simulink model "sysgenQAMExt"  (Simulink 7.7)
settings: Solver=ode45  StartTime=0.0  StopTime=3000  RelTol=1e-3
PreLoadFcn:
  | xlrequire('PreLoadFcn')
values from neighbouring files (symbols this model uses):
  hh = hh1/max(hh1)    [sysgenCostasLoop_PreLoadFcn.m]
  j = find(xLabel==')')    [sdspfscope2_r13.m]
  k = (k-1)*3+2    [sdspfscope2_r13.m]
  mu = xfix({xlSigned, 18, 15, xlRound, xlSaturate}, mu)    [lmsErr.m]
undefined symbols (not defined in the file or in its folder): chan, k_i0, k_p0, xlipgetpartsetting, xlsfunxy
libraries: xbsIndex_r4 x477, simulink x2, dspsigops x2, dspmlti4 x2, commchan3 x1, xbsCopyrightNotice_r4 x1, dspobslib x1
(part 1 of 5)
settings Model: Creator=alexc  LastModifiedBy=wayneh  ExtModeTrigMode=oneshot  ExtModeArmWhenConnect=off
settings DataIOCC: LimitDataPoints=off  SignalLoggingName=sigsOut
settings OptimizationCC: BlockReduction=off  BooleanDataType=off  InlineInvariantSignals=on  InitFltsAndDblsToZero=on
settings DebuggingCC: SaveWithParameterizedLinksMsg=none  SignalResolutionControl=TryResolveAllWithWarning  SolverPrmCheckMsg=none  MultiTaskDSMMsg=warning  MultiTaskCondExecSysMsg=none  StrictBusMsg=None
settings HardwareCC: TargetUnknown=on
settings RTWCC: IncludeERTFirstTime=on
settings GRTTargetCC: TargetFcnLib=ansi_tfl_tmw.mat

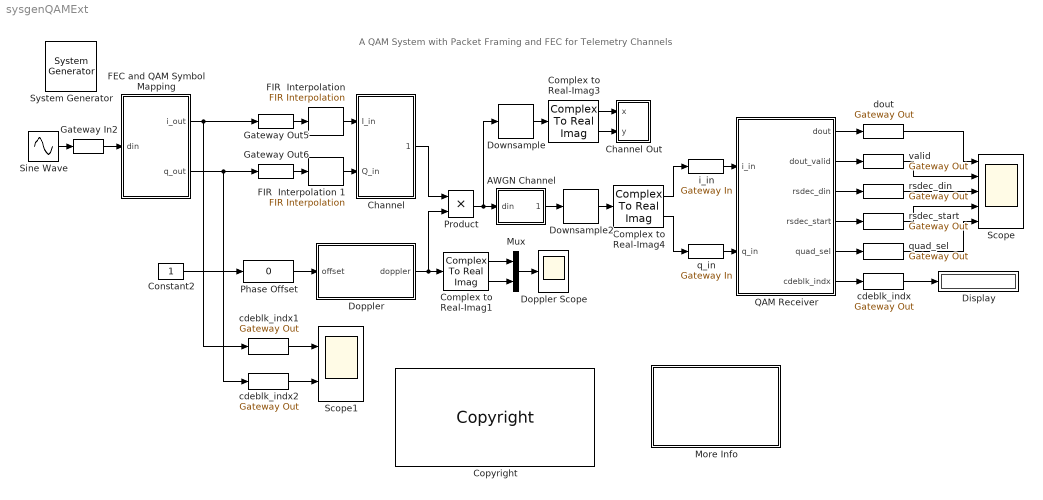
== system sysgenQAMExt ==
  note: A QAM System with Packet Framing and FEC for Telemetry Channels
  " System Generator" : xbsIndex_r4/ System Generator  Tag=genX  SystemSampleTime=-1  xilinxfamily=virtex6  part=xc6vlx240t  speed=-1  package=ff1156  synthesis_tool=XST  clock_wrapper=Clock Enables  directory=./netlist1  proj_type=Project Navigator  Synth_file=XST Defaults  Impl_file=ISE Defaults  testbench=off  simulink_period=1  sysclk_period=55  dcm_input_clock_period=100  incr_netlist=off  trim_vbits=Everywhere in SubSystem  dbl_ovrd=According to Block Masks  core_generation=According to Block Masks  run_coregen=off  deprecated_control=off  eval_field=0  block_type=sysgen
      settings: block_version=10.1.3
  AWGN Channel : Subsystem  mask{snr=4}
  Channel : Subsystem
  Channel Out : Subsystem  LoadFcn=xlsfunxy([],[],[],'LoadBlock')  StartFcn=xlsfunxy([],[],[],'Start')  StopFcn=xlsfunxy([],[],[],'Stop')  mask(My XY scope.){xmin=-2.25, xmax=2.25, ymin=-2.25, ymax=2.25, refresh=800, style='.', st=-1}
      mask prompts: xmin "x-min:"; xmax "x-max:"; ymin "y-min:"; ymax "y-max:"; refresh "Refresh rate"; style "Line/Marker style"; st "Sample time:"
      mask help: XY scope using MATLAB graph window. First input is used as time base. Enter plotting ranges.
      settings: CopyFcn=xlsfunxy([],[],[],'CopyBlock')  DeleteFcn=xlsfunxy([],[],[],'DeleteBlock')  NameChangeFcn=xlsfunxy([],[],[],'NameChange')
      mask Help: This block can be used to explore limit cycles. Look at the m-file xlsfunxy.m to see how it works.
      mask Display: plot([.05 .95 .95 .05 .05],[.45 .45 .95 .95 .45], 0.5+cos(0:0.1:2*pi)*0.3,0.7+sin(0:0.1:2*pi)*0.2)
  Complex to Real-Imag1 : ComplexToRealImag
  Complex to Real-Imag3 : ComplexToRealImag
  Complex to Real-Imag4 : ComplexToRealImag
  Constant2 : Constant
  Copyright : xbsCopyrightNotice_r4/Copyright  copyrighttext="Copyright (c) 2011  by  Xilinx, Inc. All rights reserved.<br><br>This file contains proprietary, confidential information of Xilinx, Inc., is distributed under license from Xilinx, Inc., and may be used, copied and/or disclosed only pursuant to the terms of a valid license agreement with Xilinx, Inc. Xilinx hereby grants you a license to use this file solely for design, simulation, implementation and creation of design files limited to Xilinx devices or technologies. Use with non-Xilinx devices or technologies is expressly prohibited and immediately terminates your license unless covered by a separate agreement.<br><br>Xilinx is providing this design, code, or information \"as-is\" solely for use in developing programs and solutions for Xilinx devices, with no obligation on the part of Xilinx to provide support. By providing this design, code, or information as one possible implementation of this feature, application or standard, Xilinx is making no representation that this implementation is free from any claims of infringement. You are responsible for obtaining any rights you may require for your implementation. Xilinx expressly disclaims any warranty whatsoever with respect to the adequacy of the implementation, including but not limited to any warranties or representations that this implementation is free from claims of infringement, implied warranties of merchantability or fitness for a particular purpose.<br><br>Xilinx products are not intended for use in life support appliances, devices, or systems. Use in such applications is expressly prohibited.<br><br>Any modifications that are made to the Source Code are done at the user's sole risk and will be unsupported.<br><br>This copyright and support notice must be retained as part of this text at all times. (c) Copyright 1995-2011 Xilinx, Inc. All rights reserved."  block_type=copyright
      settings: block_version=10.1.00
      settings: infoedit=|
      | Copyright(C) 2008 by  Xilinx, Inc. All rights reserved.<br>
      | <br>
      | This file contains proprietary, confidential information of Xilinx, Inc., is distributed under license
      | from Xilinx, Inc., and may be used, copied and/or disclosed only pursuant to the terms of a valid license
      | agreement with Xilinx, Inc. Xilinx hereby grants you a license to use this file solely for design,
      | simulation, implementation and creation of design files limited to Xilinx devices or technologies. Use
      | with non-Xilinx devices or technologies is expressly prohibited and immediately terminates your license
      | unless covered by a separate agreement.<br>
      | <br>
      | Xilinx is providing this design, code, or information "as-is" solely for use in developing programs and
      | solutions for Xilinx devices, with no obligation on the part of Xilinx to provide support. By providing
      | this design, code, or information as one possible implementation of this feature, application or standard,
      | Xilinx is making no representation that this implementation is free from any claims of infringement. You
      | are responsible for obtaining any rights you may require for your implementation. Xilinx expressly disclaims
      | any warranty whatsoever with respect to the adequacy of the implementation, including but not limited to any
      | warranties or representations that this implementation is free from claims of infringement, implied warranties
      | of merchantability or fitness for a particular purpose.<br>
      | <br>
      | Xilinx products are not intended for use in life support appliances, devices, or systems. Use in such
      | applications is expressly prohibited.<br>
      | <br>
      | Any modifications that are made to the Source Code are done at the user's sole risk and will be unsupported.<br>
      | <br>
      | This copyright and support notice must be retained as part of this text at all times.
      | (c) Copyright 1995-2008 Xilinx, Inc. All rights reserved.
  Display : Display
  Doppler : Subsystem
  Doppler Scope : Scope
      settings: TimeRange=4000  YMin=-0.6  YMax=1
  Downsample : dspsigops/Downsample  N=4  phase=0  InputProcessing=Inherited (this choice will be removed - see release notes)  RateOptions=Enforce single-rate processing  smode=Allow multirate  fmode=Maintain input frame size  ic=0
  Downsample2 : dspsigops/Downsample  N=2  phase=0  InputProcessing=Inherited (this choice will be removed - see release notes)  RateOptions=Enforce single-rate processing  smode=Allow multirate  fmode=Maintain input frame size  ic=0
  FEC and QAM Symbol Mapping : Subsystem
  "FIR  Interpolation " : dspmlti4/FIR Interpolation  h=[hh]  L=4  framing=Maintain input frame size  outputBufInitCond=0  InputProcessing=Inherited (this choice will be removed - see release notes)  firstCoeffDataTypeStr=Inherit: Same word length as input  firstCoeffLastDataTypeStr=Inherit: Same word length as input  firstCoeffMin=[]  firstCoeffMax=[]  outputDataTypeStr=Inherit: Same as accumulator  outputLastDataTypeStr=Inherit: Same as accumulator  outputMin=[]  outputMax=[]  roundingMode=Floor  overflowMode=off  FilterSource=Specify via dialog  FilterObject=Hm_firinterp
  FIR  Interpolation 1 : dspmlti4/FIR Interpolation  h=[hh]  L=4  framing=Maintain input frame size  outputBufInitCond=0  InputProcessing=Inherited (this choice will be removed - see release notes)  firstCoeffDataTypeStr=Inherit: Same word length as input  firstCoeffLastDataTypeStr=Inherit: Same word length as input  firstCoeffMin=[]  firstCoeffMax=[]  outputDataTypeStr=Inherit: Same as accumulator  outputLastDataTypeStr=Inherit: Same as accumulator  outputMin=[]  outputMax=[]  roundingMode=Floor  overflowMode=off  FilterSource=Specify via dialog  FilterObject=Hm_firinterp
  Gateway In2 : xbsIndex_r4/Gateway In  gui_display_data_type=Fixed-point  arith_type="Signed  (2's comp)"  n_bits=8  bin_pt=7  preci_type=Single  exp_width=8  frac_width=24  quantization="Round  (unbiased: +/- Inf)"  overflow=Saturate  period=16  dbl_ovrd=off  timing_constraint=None  locs_specified=off  LOCs={}  inherit_from_input=off  UseAsADC=off  ADCChannel='1'  hdl_port=on  block_type=gatewayin
      settings: infoedit="Gateway in block.  Converts inputs of type Simulink integer, double and fixed point to  Xilinx fixed point type.<P><P>Hardware notes:  In hardware these blocks become top level input ports."  xl_area=[0, 0, 0, 0, 0, 0, 0]  block_version=VER_STRING_GOES_HERE
  Gateway Out5 : xbsIndex_r4/Gateway Out  inherit_from_input=off  hdl_port=on  timing_constraint=None  locs_specified=off  LOCs={}  UseAsDAC=off  DACChannel='1'  block_type=gatewayout
      settings: infoedit="Gateway out block.  Converts Xilinx fixed point inputs into ouputs of type Simulink integer, double, or fixed point.<P><P>Hardware notes:  In hardware these blocks become top level output ports or are discarded, depending on how they are configured."  xl_area=[0, 0, 0, 0, 0, 0, 0]  block_version=VER_STRING_GOES_HERE
  Gateway Out6 : xbsIndex_r4/Gateway Out  inherit_from_input=off  hdl_port=on  timing_constraint=None  locs_specified=off  LOCs={}  UseAsDAC=off  DACChannel='1'  block_type=gatewayout
      settings: infoedit="Gateway out block.  Converts Xilinx fixed point inputs into ouputs of type Simulink integer, double, or fixed point.<P><P>Hardware notes:  In hardware these blocks become top level output ports or are discarded, depending on how they are configured."  xl_area=[0, 0, 0, 0, 0, 0, 0]  block_version=VER_STRING_GOES_HERE
  More Info : Subsystem
      mask Display: disp('Double click\n for\n more information.')
  Mux : Mux  Inputs=2
  Phase Offset : simulink/Math Operations/Slider Gain  SystemSampleTime=-1  low=0  gain=0  high=1
  Product : Product  SaturateOnIntegerOverflow=on  InputSameDT=on  OutDataTypeStr=Inherit: Same as first input
  QAM Receiver : Subsystem
  Scope : Scope  NumInputPorts=5
      settings: TimeRange=5000  YMin=-1~-1~-1~-1~-1  YMax=1~1~1~1~1
  Scope1 : Scope  NumInputPorts=2
      settings: TimeRange=10000  YMin=-1~-1  YMax=1~1  SaveName=ScopeData2
  Sine Wave : Sin  Frequency=1/255  SampleTime=16
  cdeblk_indx : xbsIndex_r4/Gateway Out  inherit_from_input=off  hdl_port=on  timing_constraint=None  locs_specified=off  LOCs={}  UseAsDAC=off  DACChannel='1'  block_type=gatewayout
      settings: infoedit="Gateway out block.  Converts Xilinx fixed point inputs into ouputs of type Simulink integer, double, or fixed point.<P><P>Hardware notes:  In hardware these blocks become top level output ports or are discarded, depending on how they are configured."  xl_area=[0, 0, 0, 0, 0, 0, 0]  block_version=VER_STRING_GOES_HERE
  cdeblk_indx1 : xbsIndex_r4/Gateway Out  inherit_from_input=off  hdl_port=off  timing_constraint=None  locs_specified=off  LOCs={}  UseAsDAC=off  DACChannel='1'  block_type=gatewayout
      settings: infoedit="Gateway out block.  Converts Xilinx fixed point inputs into ouputs of type Simulink integer, double, or fixed point.<br><br>Hardware notes:  In hardware these blocks become top level output ports or are discarded, depending on how they are configured."  xl_area=[0, 0, 0, 0, 0, 0, 0]  block_version=VER_STRING_GOES_HERE
  cdeblk_indx2 : xbsIndex_r4/Gateway Out  inherit_from_input=off  hdl_port=off  timing_constraint=None  locs_specified=off  LOCs={}  UseAsDAC=off  DACChannel='1'  block_type=gatewayout
      settings: infoedit="Gateway out block.  Converts Xilinx fixed point inputs into ouputs of type Simulink integer, double, or fixed point.<br><br>Hardware notes:  In hardware these blocks become top level output ports or are discarded, depending on how they are configured."  xl_area=[0, 0, 0, 0, 0, 0, 0]  block_version=VER_STRING_GOES_HERE
  dout : xbsIndex_r4/Gateway Out  inherit_from_input=off  hdl_port=on  timing_constraint=None  locs_specified=off  LOCs={}  UseAsDAC=off  DACChannel='1'  block_type=gatewayout
      settings: infoedit="Gateway out block.  Converts Xilinx fixed point inputs into ouputs of type Simulink integer, double, or fixed point.<P><P>Hardware notes:  In hardware these blocks become top level output ports or are discarded, depending on how they are configured."  xl_area=[0, 0, 0, 0, 0, 0, 0]  block_version=VER_STRING_GOES_HERE
  i_in : xbsIndex_r4/Gateway In  gui_display_data_type=Fixed-point  arith_type="Signed  (2's comp)"  n_bits=xn_ni  bin_pt=xn_nf  preci_type=Single  exp_width=8  frac_width=24  quantization="Round  (unbiased: +/- Inf)"  overflow=Saturate  period=2  dbl_ovrd=off  timing_constraint=None  locs_specified=off  LOCs={}  inherit_from_input=off  UseAsADC=off  ADCChannel='1'  hdl_port=on  block_type=gatewayin
      settings: infoedit="Gateway in block.  Converts inputs of type Simulink integer, double and fixed point to  Xilinx fixed point type.<P><P>Hardware notes:  In hardware these blocks become top level input ports."  xl_area=[0, 0, 0, 0, 0, 0, 0]  block_version=VER_STRING_GOES_HERE
  q_in : xbsIndex_r4/Gateway In  gui_display_data_type=Fixed-point  arith_type="Signed  (2's comp)"  n_bits=xn_ni  bin_pt=xn_nf  preci_type=Single  exp_width=8  frac_width=24  quantization="Round  (unbiased: +/- Inf)"  overflow=Saturate  period=2  dbl_ovrd=off  timing_constraint=None  locs_specified=off  LOCs={}  inherit_from_input=off  UseAsADC=off  ADCChannel='1'  hdl_port=on  block_type=gatewayin
      settings: infoedit="Gateway in block.  Converts inputs of type Simulink integer, double and fixed point to  Xilinx fixed point type.<P><P>Hardware notes:  In hardware these blocks become top level input ports."  xl_area=[0, 0, 0, 0, 0, 0, 0]  block_version=VER_STRING_GOES_HERE
  quad_sel : xbsIndex_r4/Gateway Out  inherit_from_input=off  hdl_port=on  timing_constraint=None  locs_specified=off  LOCs={}  UseAsDAC=off  DACChannel='1'  block_type=gatewayout
      settings: infoedit="Gateway out block.  Converts Xilinx fixed point inputs into ouputs of type Simulink integer, double, or fixed point.<P><P>Hardware notes:  In hardware these blocks become top level output ports or are discarded, depending on how they are configured."  xl_area=[0, 0, 0, 0, 0, 0, 0]  block_version=VER_STRING_GOES_HERE
  rsdec_din : xbsIndex_r4/Gateway Out  inherit_from_input=off  hdl_port=on  timing_constraint=None  locs_specified=off  LOCs={}  UseAsDAC=off  DACChannel='1'  block_type=gatewayout
      settings: infoedit="Gateway out block.  Converts Xilinx fixed point inputs into ouputs of type Simulink integer, double, or fixed point.<P><P>Hardware notes:  In hardware these blocks become top level output ports or are discarded, depending on how they are configured."  xl_area=[0, 0, 0, 0, 0, 0, 0]  block_version=VER_STRING_GOES_HERE
  rsdec_start : xbsIndex_r4/Gateway Out  inherit_from_input=off  hdl_port=on  timing_constraint=None  locs_specified=off  LOCs={}  UseAsDAC=off  DACChannel='1'  block_type=gatewayout
      settings: infoedit="Gateway out block.  Converts Xilinx fixed point inputs into ouputs of type Simulink integer, double, or fixed point.<P><P>Hardware notes:  In hardware these blocks become top level output ports or are discarded, depending on how they are configured."  xl_area=[0, 0, 0, 0, 0, 0, 0]  block_version=VER_STRING_GOES_HERE
  valid : xbsIndex_r4/Gateway Out  inherit_from_input=off  hdl_port=on  timing_constraint=None  locs_specified=off  LOCs={}  UseAsDAC=off  DACChannel='1'  block_type=gatewayout
      settings: infoedit="Gateway out block.  Converts Xilinx fixed point inputs into ouputs of type Simulink integer, double, or fixed point.<P><P>Hardware notes:  In hardware these blocks become top level output ports or are discarded, depending on how they are configured."  xl_area=[0, 0, 0, 0, 0, 0, 0]  block_version=VER_STRING_GOES_HERE
  wires:
  FEC and QAM Symbol Mapping/1(i_out) -> Gateway Out5/1, cdeblk_indx1/1
  FEC and QAM Symbol Mapping/2(q_out) -> Gateway Out6/1, cdeblk_indx2/1
  Channel/1(chan_out) -> Product/1
  Doppler/1(doppler) -> Product/2, Complex to Real-Imag1/1
  i_in/1 -> QAM Receiver/1(i_in)
  q_in/1 -> QAM Receiver/2(q_in)
  Product/1 -> AWGN Channel/1(din), Downsample/1
  Phase Offset/1 -> Doppler/1(offset)
  Constant2/1 -> Phase Offset/1
  Mux/1 -> Doppler Scope/1
  Complex to Real-Imag1/1 -> Mux/1
  Complex to Real-Imag1/2 -> Mux/2
  cdeblk_indx/1 -> Display/1
  QAM Receiver/6(cdeblk_indx) -> cdeblk_indx/1
  Downsample2/1 -> Complex to Real-Imag4/1
  Complex to Real-Imag4/2 -> q_in/1
  Complex to Real-Imag4/1 -> i_in/1
  Downsample/1 -> Complex to Real-Imag3/1
  Complex to Real-Imag3/2 -> Channel Out/2(y)
  Complex to Real-Imag3/1 -> Channel Out/1(x)
  "FIR  Interpolation "/1 -> Channel/1(I_in)
  FIR  Interpolation 1/1 -> Channel/2(Q_in)
  Gateway Out5/1 -> "FIR  Interpolation "/1
  Gateway Out6/1 -> FIR  Interpolation 1/1
  Sine Wave/1 -> Gateway In2/1
  Gateway In2/1 -> FEC and QAM Symbol Mapping/1(din)
  AWGN Channel/1(dout) -> Downsample2/1
  QAM Receiver/1(dout) -> dout/1
  QAM Receiver/2(dout_valid) -> valid/1
  QAM Receiver/3(rsdec_din) -> rsdec_din/1
  QAM Receiver/5(quad_sel) -> quad_sel/1
  QAM Receiver/4(rsdec_start) -> rsdec_start/1
  quad_sel/1 -> Scope/5
  rsdec_din/1 -> Scope/3
  rsdec_start/1 -> Scope/4
  dout/1 -> Scope/1
  valid/1 -> Scope/2
  cdeblk_indx1/1 -> Scope1/1
  cdeblk_indx2/1 -> Scope1/2

== system sysgenQAMExt/AWGN Channel ==
  din : Inport
  AWGN Channel : commchan3/AWGN Channel  SystemSampleTime=-1  InputProcessing=Inherited (this choice will be removed - see release notes)  seed=54321  noiseMode="Signal to noise ratio  (SNR)"  EbNodB=10  EsNodB=10  SNRdB=snr  bitsPerSym=1  Ps=1/16  Tsym=1  variance=1
  dout : Outport
  wires:
  AWGN Channel/1 -> dout/1
  din/1 -> AWGN Channel/1

== system sysgenQAMExt/Channel ==
  I_in : Inport
  Q_in : Inport  Port=2
  Channel : Subsystem
  Channel1 : Subsystem
  Gain : Gain  Gain=j  SaturateOnIntegerOverflow=on  OutDataTypeStr=Inherit: Same as input  ParamDataTypeStr=Inherit: Same as input
  Sum : Sum  SaturateOnIntegerOverflow=on  InputSameDT=on  OutDataTypeStr=Inherit: Same as first input
  chan_out : Outport
  wires:
  Gain/1 -> Sum/2
  Channel/1(y_n) -> Sum/1
  Channel1/1(y_n) -> Gain/1
  I_in/1 -> Channel/1(x_n)
  Q_in/1 -> Channel1/1(x_n)
  Sum/1 -> chan_out/1

== system sysgenQAMExt/Channel Out ==
  x : Inport
  y : Inport  Port=2
  Mux : Mux  Inputs=2
  xlsfunxy : S-Function  FunctionName=xlsfunxy  Parameters=[xmin xmax ymin ymax],refresh,style,st  EnableBusSupport=off
  wires:
  Mux/1 -> xlsfunxy/1
  x/1 -> Mux/1
  y/1 -> Mux/2

== system sysgenQAMExt/Doppler ==
  offset : Inport
  DSP Constant : dspobslib/DSP Constant  SystemSampleTime=-1  Value=1  SampleMode=Discrete  discreteOutput=Sample-based  continuousOutput=Sample-based  sampTime=1  framePeriod=1  dataType=Inherit from 'Constant value'  isSigned=on  wordLen=16  udDataType=sfix(16)  fracBitsMode=Best precision  numFracBits=15  InterpretAs1D=off  Ts=1  FramebasedOutput=off
  Frequency Delta : simulink/Math Operations/Slider Gain  SystemSampleTime=-1  low=-0.1  gain=0.001  high=0.1
  R:I : RealImagToComplex
  TX Doppler : Subsystem
  Terminator : Terminator
  doppler : Outport
  wires:
  TX Doppler/1(Cos) -> R:I/1
  TX Doppler/2(Sin) -> R:I/2
  DSP Constant/1 -> Frequency Delta/1
  R:I/1 -> doppler/1
  TX Doppler/3(DDS Theta) -> Terminator/1
  Frequency Delta/1 -> TX Doppler/1(In1)
  offset/1 -> TX Doppler/2(Phase Offset)

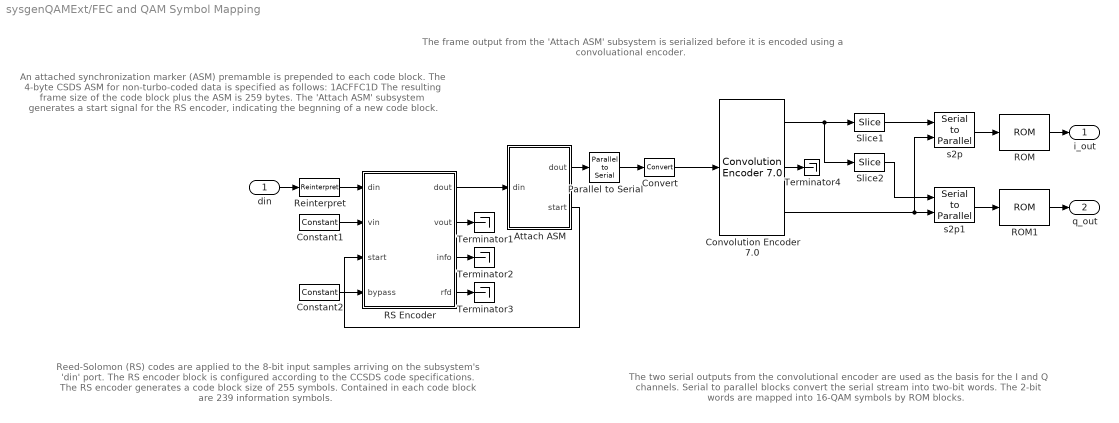
== system sysgenQAMExt/FEC and QAM Symbol Mapping ==
  note: Reed-Solomon (RS) codes are applied to the 8-bit input samples
      | arriving on the subsystem's 'din' port.  The RS encoder block is
      | configured according to the CCSDS code specifications.  The RS
      | encoder generates a code block size of 255 symbols.  Contained
      | in each code block are 239 information symbols.
  note: An attached synchronization marker (ASM) premamble
      | is prepended to each code block.  The 4-byte CSDS
      | ASM for non-turbo-coded data is specified as follows:
      |
      | 1ACFFC1D
      |
      | The resulting frame size of the code block plus the ASM
      | is  259 bytes.  The 'Attach ASM' subsystem generates a
      | start signal for the RS encoder, indicating the begnning
      | of a new code block.
  note: The frame output from the 'Attach ASM' subsystem is serialized
      | before it is encoded using a convoluational encoder.
  note: The two serial outputs from the convolutional
      | encoder are used as the basis for the I and Q
      | channels.  Serial to parallel blocks convert the
      | serial stream into two-bit words.
      |
      | The 2-bit words are mapped into 16-QAM
      | symbols by ROM blocks.
  din : Inport
  Attach ASM : Subsystem
  Constant1 : xbsIndex_r4/Constant  const=1  gui_display_data_type=Fixed-point  arith_type=Boolean  n_bits=1  bin_pt=0  preci_type=Single  exp_width=8  frac_width=24  explicit_period=off  period=1  equ=P=C  opselect=C  inp2=PCIN>>17  opr=+  inp1=P  carry=CIN  dbl_ovrd=off  block_type=constant
      settings: block_version=VER_STRING_GOES_HERE
  Constant2 : xbsIndex_r4/Constant  const=0  gui_display_data_type=Fixed-point  arith_type=Boolean  n_bits=1  bin_pt=0  preci_type=Single  exp_width=8  frac_width=24  explicit_period=off  period=1  equ=P=C  opselect=C  inp2=PCIN>>17  opr=+  inp1=P  carry=CIN  dbl_ovrd=off  block_type=constant
      settings: block_version=VER_STRING_GOES_HERE
  Convert : xbsIndex_r4/Convert  gui_display_data_type=Fixed-point  arith_type=Boolean  n_bits=16  bin_pt=14  float_type=Single  exp_bits=8  fraction_bits=24  quantization=Truncate  overflow=Wrap  en=off  latency=0  dbl_ovrd=off  pipeline=off  block_type=convert
      settings: block_version=11.4
  "Convolution Encoder 7.0 " : xbsIndex_r4/Convolution Encoder 7.0   input_rate=1  output_rate=2  punctured=off  dual_output=off  puncture_code0='0'  puncture_code1='0'  constraint_length=7  convolution_code0='1111001'  convolution_code1='1011011'  convolution_code2='0000011'  convolution_code3='0000011'  convolution_code4='0000011'  convolution_code5='0000011'  convolution_code6='0000011'  nd=off  rfd=on  fd_in=off  rffd=off  rdy=on  synchronous_clear=off  ce=off  ip_name=Convolution Encoder  ip_version=7.0  dsptool_ready=false  ipcore_usecache=true  ipcore_useipmodelcache=true  wrapper_available=true  port_translation_map={ 'ce' => 'en', 'sclr' => 'rst'}  structural_sim=true  ipcore_do_not_force_period=true  block_type=convolution_v7_0
      settings: block_version=11.4
  Parallel to Serial : xbsIndex_r4/Parallel to Serial  output_order=Most Significant Word First  arith_type=Unsigned  output_bits=1  bin_pt=0  rst=off  en=off  latency=0  dbl_ovrd=off  block_type=p2s
      settings: infoedit=Each sample presented at the input becomes several samples presented serially at the output.  xl_area=[0, 0, 0, 0, 0, 0, 0]  block_version=VER_STRING_GOES_HERE
  ROM : xbsIndex_r4/ROM  depth=4  initVector=[1/3 1 -1/3 -1]  distributed_mem=Block RAM  rst=off  init_reg=0  en=off  latency=1  gui_display_data_type=Fixed-point  arith_type="Signed  (2's comp)"  n_bits=16  bin_pt=15  preci_type=Single  exp_width=8  frac_width=24  dbl_ovrd=off  optimize=Area  use_rpm=off  block_type=sprom
      settings: xl_area=[0, 0, 0, 0, 0, 0, 0]  block_version=VER_STRING_GOES_HERE
  ROM1 : xbsIndex_r4/ROM  depth=4  initVector=[1/3 1 -1/3 -1]  distributed_mem=Block RAM  rst=off  init_reg=0  en=off  latency=1  gui_display_data_type=Fixed-point  arith_type="Signed  (2's comp)"  n_bits=16  bin_pt=15  preci_type=Single  exp_width=8  frac_width=24  dbl_ovrd=off  optimize=Area  use_rpm=off  block_type=sprom
      settings: xl_area=[0, 0, 0, 0, 0, 0, 0]  block_version=VER_STRING_GOES_HERE
  RS Encoder : Subsystem
      settings: CopyFcn=set_param(gcb, 'LinkStatus', 'none');
  Reinterpret : xbsIndex_r4/Reinterpret  force_arith_type=on  arith_type=Unsigned  force_bin_pt=on  bin_pt=0  block_type=cast
      settings: infoedit="Changes type of samples without altering their binary representation.<P><P>Hardware notes: In hardware this block costs nothing.<P><P>Example:  Suppose the input is 6 bits wide, signed, with 2 fractional bits, and the output is forced to unsigned with 0 fractional bits.  Then an input of -2.0 (1110.00 in binary 2's complement) becomes an output of 56 (111000 in binary)."  block_version=VER_STRING_GOES_HERE
  Slice1 : xbsIndex_r4/Slice  nbits=1  boolean_output=off  mode=Lower Bit Location + Width  bit1=0  base1=MSB of Input  bit0=0  base0=LSB of Input  dbl_ovrd=off  block_type=slice
  Slice2 : xbsIndex_r4/Slice  nbits=1  boolean_output=off  mode=Upper Bit Location + Width  bit1=0  base1=MSB of Input  bit0=0  base0=LSB of Input  dbl_ovrd=off  block_type=slice
  Terminator{1..4} (4 alike) : Terminator
  s2p : xbsIndex_r4/Serial to Parallel  input_order=Least Significant Word First  arith_type=Unsigned  output_bits=2  bin_pt=0  rst=off  en=on  latency=1  dbl_ovrd=off  block_type=s2p
      settings: infoedit=Groups of samples presented serially at the input become single samples presented at the output.  xl_area=[0, 0, 0, 0, 0, 0, 0]  block_version=VER_STRING_GOES_HERE
  s2p1 : xbsIndex_r4/Serial to Parallel  input_order=Least Significant Word First  arith_type=Unsigned  output_bits=2  bin_pt=0  rst=off  en=on  latency=1  dbl_ovrd=off  block_type=s2p
      settings: infoedit=Groups of samples presented serially at the input become single samples presented at the output.  xl_area=[0, 0, 0, 0, 0, 0, 0]  block_version=VER_STRING_GOES_HERE
  i_out : Outport
  q_out : Outport  Port=2
  wires:
  ROM/1 -> i_out/1
  ROM1/1 -> q_out/1
  "Convolution Encoder 7.0 "/1 -> Slice1/1, Slice2/1
  s2p/1 -> ROM/1
  s2p1/1 -> ROM1/1
  Parallel to Serial/1 -> Convert/1
  Attach ASM/1(dout) -> Parallel to Serial/1
  din/1 -> Reinterpret/1
  RS Encoder/1(dout) -> Attach ASM/1(din)
  Constant1/1 -> RS Encoder/2(vin)
  Constant2/1 -> RS Encoder/4(bypass)
  Attach ASM/2(start) -> RS Encoder/3(start)
  Reinterpret/1 -> RS Encoder/1(din)
  RS Encoder/2(vout) -> Terminator1/1
  RS Encoder/3(info) -> Terminator2/1
  RS Encoder/4(rfd) -> Terminator3/1
  Convert/1 -> "Convolution Encoder 7.0 "/1
  Slice1/1 -> s2p/1
  Slice2/1 -> s2p1/1
  "Convolution Encoder 7.0 "/3 -> s2p1/2, s2p/2
  "Convolution Encoder 7.0 "/2 -> Terminator4/1

== system sysgenQAMExt/More Info ==
  note: A QAM System with Packet Framing and FEC for Telemetry Channels
  note: This design implements a QAM system with packet framing and FEC for telemetry channels.
      | The system is implemented according to the specifications provided by the Consultative
      | Committee for Space Data Systems for telemetry channel coding specification
      | (CCSDS 101.0-B-5).
      |
      | A sinusoidal source provides 8-bit samples to the 'FEC and QAM Symbol Mapping' subsystem.
      | Forward Error Correction (FEC) is applied to the samples and an attached synchronization
      | marker (ASM) is asserted at the start of each code block.   The data is mapped into 16-QAM
      | symbols and then interpolated.  Doppler content, ISI, and white Guassian noise are introduced
      | into the signal before it enters the receiver subsystem.
      |
      | The receiver employs a 16-QAM demodulator that performs adaptive channel equalization
      | and carrier recovery on a QAM input source.  The ASM is stripped from the demodulated data
      | before concatenated FEC is applied.  A PicoBlaze microcontroller controls the RS decoder,
      | maintains frame alignment of the received packects, and performs periodic adjustments of
      | the de-mapping QAM-16 quadrant reference.
      |
      | The CCSDS specification document can be found at the following URL:
      | http://nssdcftp.gsfc.nasa.gov/standards/ccsds/pdf/CCSDS-101.0-B-5.pdf
      |
      | For more information on the 16-QAM demodulator implementation and FPGA software-defined radios
      | in general, consult the following references:
      |
      | Chris H. Dick and Fred Harris, "FPGA QAM Demodulator Design," Field Programmable Logic
      | Conference (FPL), Sept. 2-4 Montpellier, France, 2002.
      |
      | Chris H. Dick, "Design and implementation of high-performance FPGA signal processing
      | datapaths for software-defined radios" VMEbus Systems, August 2001

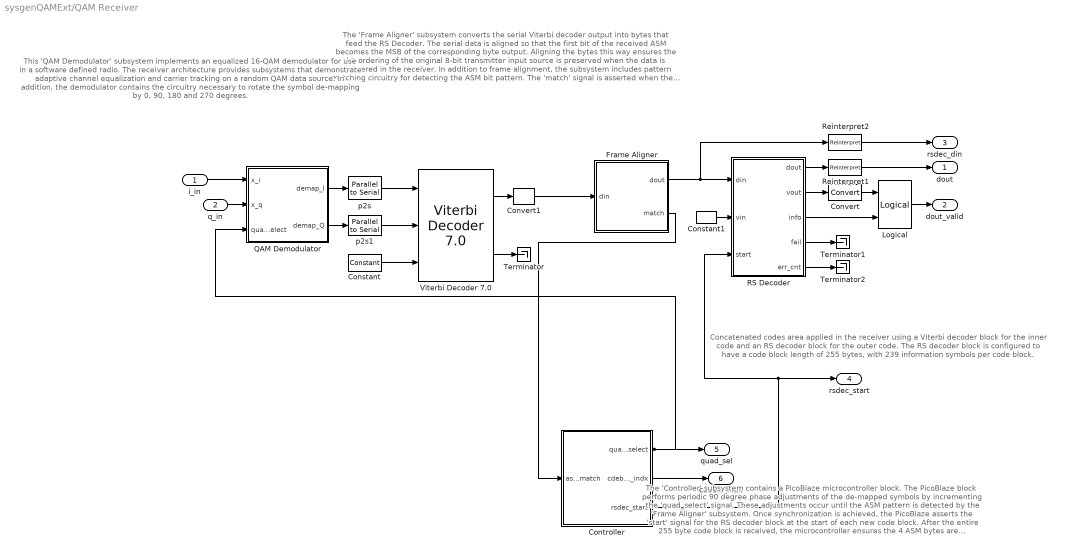
== system sysgenQAMExt/QAM Receiver ==
  note: The 'Frame Aligner' subsystem converts the serial Viterbi decoder output
      | into bytes that feed the RS Decoder.  The serial data is aligned so that the
      | first bit of the received ASM  becomes the MSB of the corresponding byte
      | output.  Aligning the bytes this way ensures the bit ordering of the original
      | 8-bit transmitter input source is preserved when the data is recovered in the
      | receiver.
      |
      | In addition to frame alignment, the subsystem includes pattern matching
      | circuitry for detecting the ASM bit pattern. The 'match' signal is asserted
      | when the ASM is detected.  The match signal is asserted when the last
      | byte of the ASM is presented on the 'dout' port.
  note: The 'Controller' subsystem contains a PicoBlaze microcontroller block.
      | The PicoBlaze block performs periodic 90 degree phase adjustments of
      | the de-mapped symbols by incrementing the 'quad_select' signal.
      | These adjustments occur until the ASM pattern is detected by the 'Frame
      | Aligner' subsystem.
      |
      | Once synchronization is achieved, the PicoBlaze asserts the 'start' signal
      | for the RS decoder block at the start of each new code block.  After the
      | entire 255 byte code block is received, the microcontroller ensures the 4
      | ASM bytes are successfully detected in the frame aligner.
      |
      | If synchronization is lost, i.e. the ASM is not detected, the microcontroller
      | will continue making adjustments to the 'quad_select' signal until the ASM
      | is once again detected.
  note: This 'QAM Demodulator' subsystem implements an equalized 16-QAM
      | demodulator for use in a software defined radio.  The receiver
      | architecture provides subsystems that demonstrate adaptive channel
      | equalization and carrier tracking on a random QAM data source.  In
      | addition, the demodulator contains the circuitry necessary to rotate the
      | symbol de-mapping by 0, 90, 180 and 270 degrees.
  note: Concatenated codes area applied in the receiver
      | using a Viterbi decoder block for the inner code
      | and an RS decoder block for the outer code.  The
      | RS decoder block is configured to have a code
      | block length of 255 bytes, with 239 information
      | symbols per code block.
  i_in : Inport
  q_in : Inport  Port=2
  Constant : xbsIndex_r4/Constant  const=1  gui_display_data_type=Fixed-point  arith_type=Boolean  n_bits=1  bin_pt=0  preci_type=Single  exp_width=8  frac_width=24  explicit_period=off  period=1  equ=P=C  opselect=C  inp2=PCIN>>17  opr=+  inp1=P  carry=CIN  dbl_ovrd=off  block_type=constant
      settings: block_version=VER_STRING_GOES_HERE
  Constant1 : xbsIndex_r4/Constant  const=1  gui_display_data_type=Fixed-point  arith_type=Boolean  n_bits=1  bin_pt=0  preci_type=Single  exp_width=8  frac_width=24  explicit_period=off  period=1  equ=P=C  opselect=C  inp2=PCIN>>17  opr=+  inp1=P  carry=CIN  dbl_ovrd=off  block_type=constant
      settings: block_version=VER_STRING_GOES_HERE
  Controller : Subsystem
  Convert : xbsIndex_r4/Convert  gui_display_data_type=Fixed-point  arith_type=Unsigned  n_bits=1  bin_pt=0  float_type=Single  exp_bits=8  fraction_bits=24  quantization=Truncate  overflow=Wrap  en=off  latency=0  dbl_ovrd=off  pipeline=off  block_type=convert
      settings: infoedit=The input is presented at the output after quantization and overflow effects.<P><P>Hardware notes: Additional hardware is used when rounding or saturation is selected and output width is less than the input width.  xl_area=[0, 0, 0, 0, 0, 0, 0]  block_version=VER_STRING_GOES_HERE
  Convert1 : xbsIndex_r4/Convert  gui_display_data_type=Fixed-point  arith_type=Unsigned  n_bits=1  bin_pt=0  float_type=Single  exp_bits=8  fraction_bits=24  quantization=Truncate  overflow=Wrap  en=off  latency=0  dbl_ovrd=off  pipeline=off  block_type=convert
      settings: block_version=11.4
  Frame Aligner : Subsystem
  Logical : xbsIndex_r4/Logical  logical_function=AND  inputs=2  en=off  latency=0  precision=Full  arith_type=Unsigned  n_bits=8  bin_pt=2  align_bp=on  dbl_ovrd=off  block_type=logical
      settings: xl_area=[0, 0, 0, 0, 0, 0, 0]  block_version=VER_STRING_GOES_HERE
  QAM Demodulator : Subsystem
  RS Decoder : Subsystem
      settings: CopyFcn=set_param(gcb, 'LinkStatus', 'none');
  Reinterpret1 : xbsIndex_r4/Reinterpret  force_arith_type=on  arith_type="Signed  (2's comp)"  force_bin_pt=on  bin_pt=7  block_type=cast
      settings: infoedit="Changes type of samples without altering their binary representation.<P><P>Hardware notes: In hardware this block costs nothing.<P><P>Example:  Suppose the input is 6 bits wide, signed, with 2 fractional bits, and the output is forced to unsigned with 0 fractional bits.  Then an input of -2.0 (1110.00 in binary 2's complement) becomes an output of 56 (111000 in binary)."  block_version=VER_STRING_GOES_HERE
  Reinterpret2 : xbsIndex_r4/Reinterpret  force_arith_type=on  arith_type="Signed  (2's comp)"  force_bin_pt=on  bin_pt=7  block_type=cast
      settings: infoedit="Changes type of samples without altering their binary representation.<P><P>Hardware notes: In hardware this block costs nothing.<P><P>Example:  Suppose the input is 6 bits wide, signed, with 2 fractional bits, and the output is forced to unsigned with 0 fractional bits.  Then an input of -2.0 (1110.00 in binary 2's complement) becomes an output of 56 (111000 in binary)."  block_version=VER_STRING_GOES_HERE
  Terminator : Terminator
  Terminator1 : Terminator
  Terminator2 : Terminator
  "Viterbi Decoder 7.0 " : xbsIndex_r4/Viterbi Decoder 7.0   channels=1  viterbi_type=Standard  reduced_latency=off  constraint_length=7  traceback_length=96  architecture=Parallel  best_state=on  best_state_width=3  soft_width=1  coding=Hard_Coding  data_format=Signed_Magnitude  output_rate0=2  convolution_code_0_radix=Binary  convolution0_code0='1111001'  convolution0_code1='1011011'  convolution0_code2='0'  convolution0_code3='0'  convolution0_code4='0'  convolution0_code5='0'  convolution0_code6='0'  output_rate1=2  convolution_code_1_radix=Binary  convolution1_code0='1111001'  convolution1_code1='1011011'  convolution1_code2='0'  convolution1_code3='0'  convolution1_code4='0'  convolution1_code5='0'  convolution1_code6='0'  trellis_initialization=None  maximum_direct=96  direct_traceback=None  puncturing=None  ber_symbol_count=off  number_of_ber_symbols=300  synchronization=off  dynamic_thresholds=off  ber_thresh=600  norm_thresh=250  ce=off  rdy=off  synchronous_clear=off  norm=off  block_valid=on  ip_name=Viterbi Decoder  ip_version=7.0  dsptool_ready=false  ipcore_usecache=true  ipcore_useipmodelcache=true  wrapper_available=true  port_translation_map={ 'ce' => 'en', 'sclr' => 'rst'}  structural_sim=false  block_type=viterbi_v7_0
      settings: block_version=11.4
  p2s : xbsIndex_r4/Parallel to Serial  output_order=Least Significant Word First  arith_type=Unsigned  output_bits=1  bin_pt=0  rst=off  en=off  latency=0  dbl_ovrd=off  block_type=p2s
      settings: infoedit=Each sample presented at the input becomes several samples presented serially at the output.  xl_area=[0, 0, 0, 0, 0, 0, 0]  block_version=VER_STRING_GOES_HERE
  p2s1 : xbsIndex_r4/Parallel to Serial  output_order=Least Significant Word First  arith_type=Unsigned  output_bits=1  bin_pt=0  rst=off  en=off  latency=0  dbl_ovrd=off  block_type=p2s
      settings: infoedit=Each sample presented at the input becomes several samples presented serially at the output.  xl_area=[0, 0, 0, 0, 0, 0, 0]  block_version=VER_STRING_GOES_HERE
  dout : Outport
  dout_valid : Outport  Port=2
  rsdec_din : Outport  Port=3
  rsdec_start : Outport  Port=4
  quad_sel : Outport  Port=5
  cdeblk_indx : Outport  Port=6
  wires:
  p2s/1 -> "Viterbi Decoder 7.0 "/1
  p2s1/1 -> "Viterbi Decoder 7.0 "/2
  QAM Demodulator/2(demap_Q) -> p2s1/1
  QAM Demodulator/1(demap_I) -> p2s/1
  Frame Aligner/2(match) -> Controller/1(asm_match)
  Frame Aligner/1(dout) -> RS Decoder/1(din), Reinterpret2/1
  Constant1/1 -> RS Decoder/2(vin)
  Controller/2(cdeblk_indx) -> cdeblk_indx/1
  RS Decoder/1(dout) -> Reinterpret1/1
  RS Decoder/5(err_cnt) -> Terminator2/1
  RS Decoder/2(vout) -> Convert/1
  i_in/1 -> QAM Demodulator/1(x_i)
  q_in/1 -> QAM Demodulator/2(x_q)
  Reinterpret1/1 -> dout/1
  Controller/1(quad_select) -> QAM Demodulator/3(quad_select), quad_sel/1
  RS Decoder/3(info) -> Logical/2
  Convert/1 -> Logical/1
  Logical/1 -> dout_valid/1
  Controller/3(rsdec_start) -> rsdec_start/1, RS Decoder/3(start)
  RS Decoder/4(fail) -> Terminator1/1
  Reinterpret2/1 -> rsdec_din/1
  "Viterbi Decoder 7.0 "/1 -> Convert1/1
  Constant/1 -> "Viterbi Decoder 7.0 "/3
  "Viterbi Decoder 7.0 "/2 -> Terminator/1
  Convert1/1 -> Frame Aligner/1(din)

== system sysgenQAMExt/Channel/Channel ==
  x_n : Inport
  Channel Response : Subsystem
  y_n : Outport
  wires:
  Channel Response/1(y_n) -> y_n/1
  x_n/1 -> Channel Response/1(x_n)

== system sysgenQAMExt/Channel/Channel1 ==
  x_n : Inport
  Channel Response : Subsystem
  y_n : Outport
  wires:
  Channel Response/1(y_n) -> y_n/1
  x_n/1 -> Channel Response/1(x_n)

== system sysgenQAMExt/Doppler/TX Doppler ==
  In1 : Inport
  Phase Offset : Inport  Port=2
  Sum : Sum  Inputs=|++  SaturateOnIntegerOverflow=on
  Sum5 : Sum  Inputs=|++  SaturateOnIntegerOverflow=on  InputSameDT=on  OutDataTypeStr=Inherit: Same as first input
  Trigonometric Function1 : Trigonometry  Operator=cos
  Trigonometric Function2 : Trigonometry
  Unit Delay2 : UnitDelay
  c2 : Gain  Gain=2*pi  SaturateOnIntegerOverflow=on  OutDataTypeStr=Inherit: Same as input  ParamDataTypeStr=Inherit: Same as input
  c3 : Gain  SaturateOnIntegerOverflow=on  OutDataTypeStr=Inherit: Same as input  ParamDataTypeStr=Inherit: Same as input
  Cos : Outport
  Sin : Outport  Port=2
  DDS Theta : Outport  Port=3
  wires:
  c2/1 -> Trigonometric Function1/1, Trigonometric Function2/1, DDS Theta/1
  Sum5/1 -> Unit Delay2/1
  Unit Delay2/1 -> Sum5/2, Sum/1
  Trigonometric Function2/1 -> c3/1
  c3/1 -> Sin/1
  Trigonometric Function1/1 -> Cos/1
  In1/1 -> Sum5/1
  Phase Offset/1 -> Sum/2
  Sum/1 -> c2/1

== system sysgenQAMExt/FEC and QAM Symbol Mapping/Attach ASM ==
  note: An addressable shift register (ASR) block, 'ASR1', is preconfigured with
      | three bytes of the attached synchronization marker (ASM).  Register block
      | 'r1' contains the most significant byte of the ASM.  The register output is
      | fed back to the ASR;  when the ASR is enabled the ASM shifts through
      | the feedback loop.
  note: A counter block, 'count1' produces a count-limited sequence from
      | 0 to 258.  A 'start' pulse is asserted when the count is reset to 0.
      | This pulse is used to drive the 'start' port of the RS encoder and
      | indicates the start of a new code block.
  note: A mux selects between output from the RS encoder and
      | the ASM signal.  The ASM signal is inserted as a premable
      | before each RS encoder codeblock.  The RS encoder has
      | an inherent latency of 7 cycles.  We consider this latency,
      | plus the fact that the 4-byte ASM must preceed the code
      | block, when we delay the ASM data and 'sel' signal by 3
      | cycles.  Registers 'r2,' 'r3,' and 'r4' are initialized with 1.
      | This allows us to filter out indeterminate data from the
      | RS encoder.
  din : Inport
  ASR1 : xbsIndex_r4/Addressable Shift Register  infer_latency=on  depth=2  initVector=[29 252 207]  en=on  dbl_ovrd=off  use_behavioral_HDL=off  Optimization=Resource  use_rpm=off  block_type=addrsr
      settings: infoedit="Delay of configurable length.  Any element in the delay line can be addressed and driven onto the output port.<P><P>Hardware notes: Implemented using SRL16s.  If a Virtex-II device is used, multiple SRLC16s are cascaded together."  xl_area=[0, 0, 0, 0, 0, 0, 0]  block_version=VER_STRING_GOES_HERE
  Constant : xbsIndex_r4/Constant  const=2  gui_display_data_type=Fixed-point  arith_type=Unsigned  n_bits=2  bin_pt=0  preci_type=Single  exp_width=8  frac_width=24  explicit_period=off  period=1  equ=P=C  opselect=C  inp2=PCIN>>17  opr=+  inp1=P  carry=CIN  dbl_ovrd=off  block_type=constant
      settings: block_version=VER_STRING_GOES_HERE
  Constant1 : xbsIndex_r4/Constant  const=4  gui_display_data_type=Fixed-point  arith_type=Unsigned  n_bits=3  bin_pt=0  preci_type=Single  exp_width=8  frac_width=24  explicit_period=off  period=1  equ=P=C  opselect=C  inp2=PCIN>>17  opr=+  inp1=P  carry=CIN  dbl_ovrd=off  block_type=constant
      settings: block_version=VER_STRING_GOES_HERE
  Constant2 : xbsIndex_r4/Constant  const=0  gui_display_data_type=Fixed-point  arith_type=Unsigned  n_bits=3  bin_pt=0  preci_type=Single  exp_width=8  frac_width=24  explicit_period=off  period=1  equ=P=C  opselect=C  inp2=PCIN>>17  opr=+  inp1=P  carry=CIN  dbl_ovrd=off  block_type=constant
      settings: block_version=VER_STRING_GOES_HERE
  Convert1 : xbsIndex_r4/Convert  gui_display_data_type=Fixed-point  arith_type=Unsigned  n_bits=8  bin_pt=0  float_type=Single  exp_bits=8  fraction_bits=24  quantization=Truncate  overflow=Wrap  en=off  latency=0  dbl_ovrd=off  pipeline=off  block_type=convert
      settings: infoedit=The input is presented at the output after quantization and overflow effects.<P><P>Hardware notes: Additional hardware is used when rounding or saturation is selected and output width is less than the input width.  xl_area=[0, 0, 0, 0, 0, 0, 0]  block_version=VER_STRING_GOES_HERE
  Mux1 : xbsIndex_r4/Mux  inputs=2  en=off  latency=0  precision=Full  arith_type="Signed  (2's comp)"  n_bits=8  bin_pt=2  quantization=Truncate  overflow=Wrap  dbl_ovrd=off  block_type=mux
      settings: xl_area=[0, 0, 0, 0, 0, 0, 0]  block_version=VER_STRING_GOES_HERE
  Reinterpret : xbsIndex_r4/Reinterpret  force_arith_type=on  arith_type=Unsigned  force_bin_pt=on  bin_pt=0  block_type=cast
      settings: infoedit="Changes type of samples without altering their binary representation.<P><P>Hardware notes: In hardware this block costs nothing.<P><P>Example:  Suppose the input is 6 bits wide, signed, with 2 fractional bits, and the output is forced to unsigned with 0 fractional bits.  Then an input of -2.0 (1110.00 in binary 2's complement) becomes an output of 56 (111000 in binary)."  block_version=VER_STRING_GOES_HERE
  Relational : xbsIndex_r4/Relational  mode=a<b  en=off  latency=0  dbl_ovrd=off  block_type=relational
      settings: xl_area=[0, 0, 0, 0, 0, 0, 0]  block_version=VER_STRING_GOES_HERE
  Relational1 : xbsIndex_r4/Relational  mode=a=b  en=off  latency=0  dbl_ovrd=off  block_type=relational
      settings: xl_area=[0, 0, 0, 0, 0, 0, 0]  block_version=VER_STRING_GOES_HERE
  count1 : xbsIndex_r4/Counter  cnt_type=Count Limited  cnt_to=258  operation=Up  start_count=0  cnt_by_val=1  arith_type=Unsigned  n_bits=9  bin_pt=0  load_pin=off  rst=off  en=off  explicit_period=off  period=16  dbl_ovrd=off  use_behavioral_HDL=off  implementation=Fabric  use_rpm=off  block_type=counter
      settings: infoedit="Configurable up, down and up/down counter.<P><P>Hardware notes: Free running counters are the least expensive in hardware.  A count limited counter is implemented by combining a counter with a comparator."  xl_area=[0, 0, 0, 0, 0, 0, 0]  block_version=VER_STRING_GOES_HERE
  d1 : xbsIndex_r4/Delay  rst=off  infoeditControl=Selection of Reset will increase slice count due to use of real FFs and instead of SRLs  en=off  latency=3  dbl_ovrd=off  reg_retiming=off  block_type=delay
      settings: infoedit="Delay line having  configurable length.<P><P>Hardware notes: A delay line is a chain, each link of which is an SRL16 followed by a flip-flop. If register retiming is enabled, the delay line is a chain of flip-flops."  xl_area=[0, 0, 0, 0, 0, 0, 0]  block_version=VER_STRING_GOES_HERE
  r1 : xbsIndex_r4/Register  init=26  rst=off  en=on  dbl_ovrd=off  block_type=register
      settings: xl_area=[0, 0, 0, 0, 0, 0, 0]  block_version=VER_STRING_GOES_HERE
  r2 : xbsIndex_r4/Register  init=1  rst=off  en=off  dbl_ovrd=off  block_type=register
      settings: xl_area=[0, 0, 0, 0, 0, 0, 0]  block_version=VER_STRING_GOES_HERE
  r3 : xbsIndex_r4/Register  init=1  rst=off  en=off  dbl_ovrd=off  block_type=register
      settings: xl_area=[0, 0, 0, 0, 0, 0, 0]  block_version=VER_STRING_GOES_HERE
  r4 : xbsIndex_r4/Register  init=1  rst=off  en=off  dbl_ovrd=off  block_type=register
      settings: xl_area=[0, 0, 0, 0, 0, 0, 0]  block_version=VER_STRING_GOES_HERE
  dout : Outport
  start : Outport  Port=2
  wires:
  count1/1 -> Relational/1, Relational1/1
  Convert1/1 -> ASR1/1
  Constant/1 -> ASR1/2
  Relational/1 -> r1/2, r2/1, ASR1/3
  ASR1/1 -> r1/1
  r1/1 -> Convert1/1, d1/1
  din/1 -> Reinterpret/1
  Mux1/1 -> dout/1
  Reinterpret/1 -> Mux1/2
  Constant1/1 -> Relational/2
  Constant2/1 -> Relational1/2
  Relational1/1 -> start/1
  d1/1 -> Mux1/3
  r4/1 -> Mux1/1
  r3/1 -> r4/1
  r2/1 -> r3/1

== system sysgenQAMExt/FEC and QAM Symbol Mapping/RS Encoder ==
  din : Inport
  vin : Inport  Port=2
  start : Inport  Port=3
  bypass : Inport  Port=4
  Delay : xbsIndex_r4/Delay  rst=off  infoeditControl=Selection of Reset will increase slice count due to use of real FFs and instead of SRLs  en=off  latency=5  dbl_ovrd=off  reg_retiming=off  block_type=delay
      settings: infoedit="Delay line having  configurable length.<P><P>Hardware notes: A delay line is a chain, each link of which is an SRL16 followed by a flip-flop. If register retiming is enabled, the delay line is a chain of flip-flops."  block_version=VER_STRING_GOES_HERE
  "Reed-Solomon Encoder 7.1 " : xbsIndex_r4/Reed-Solomon Encoder 7.1   code_specification=CCSDS  variable_number_of_check_symbols=off  variable_block_length=off  symbol_width=8  field_polynomial=391  scaling_factor=1  generator_start=0  symbol_per_block=255  data_symbols=239  check_symbol_generator=Fixed_Architecture  memory_style=Automatic  number_of_channels=1  ce=off  rdy=on  nd=on  rfd=on  sclr=off  rffd=off  ip_name=Reed-Solomon Encoder  ip_version=7.1  dsptool_ready=false  ipcore_usecache=true  ipcore_useipmodelcache=true  wrapper_available=true  port_translation_map={ 'ce' => 'en', 'sclr' => 'rst'}  structural_sim=false  ipcore_do_not_force_period=true  block_type=rs_encoder_v7_1
  Subsystem1 : Subsystem
  Subsystem2 : Subsystem
  dout : Outport
  vout : Outport  Port=2
  info : Outport  Port=3
  rfd : Outport  Port=4
  wires:
  Subsystem2/1(const) -> Delay/1
  din/1 -> "Reed-Solomon Encoder 7.1 "/1
  "Reed-Solomon Encoder 7.1 "/1 -> dout/1
  "Reed-Solomon Encoder 7.1 "/2 -> info/1
  bypass/1 -> "Reed-Solomon Encoder 7.1 "/2
  vin/1 -> "Reed-Solomon Encoder 7.1 "/4
  start/1 -> Subsystem2/1(sample), "Reed-Solomon Encoder 7.1 "/3
  "Reed-Solomon Encoder 7.1 "/3 -> Subsystem1/1(ufix_vout)
  "Reed-Solomon Encoder 7.1 "/4 -> Subsystem1/2(ufix_rfd)
  Subsystem1/2(bool_rfd) -> rfd/1
  Subsystem1/1(bool_vout) -> vout/1
  Delay/1 -> Subsystem1/3(sel)
